simulink model "ABS_demo"  (R2018a)
settings: Solver=ode23t  StartTime=0.0  StopTime=20  RelTol=1e-3
values from neighbouring files (symbols this model uses):
  g = 9.81    [variables_values.m]
  I = 5    [variables_values.m]
  m = 75    [variables_values.m]
  R = 1.25    [variables_values.m]
  v0 = 44    [variables_values.m]
libraries: simulink x3
settings Model: Creator=Stephen Kingston  LastModifiedBy=adham
settings DataIOCC: ReturnWorkspaceOutputs=on
settings SFSimCC: SimUseLocalCustomCode=on
settings RTWCC: RTWUseLocalCustomCode=on

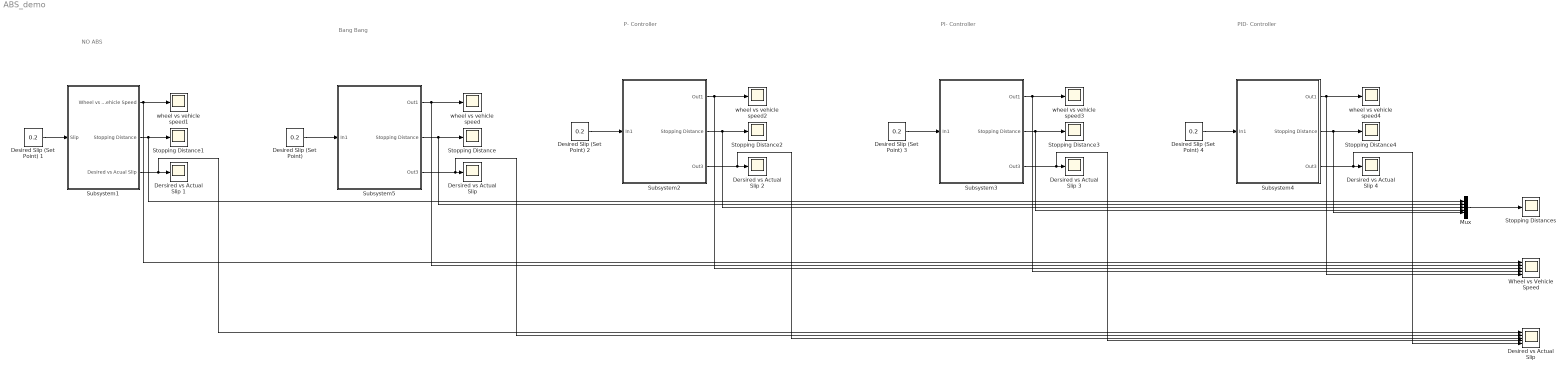
== system ABS_demo ==
  note: NO ABS
  note: Bang Bang
  note: P- Controller
  note: PI- Controller
  note: PID- Controller
  Dersired vs Actual Slip {,1..4} (5 alike) : Scope
  Desired Slip (Set Point) {,1..4} (5 alike) : Constant  Value=0.2
  Desired vs Actual Slip : Scope  NumInputPorts=5
  Mux : Mux  Inputs=5
  Stopping Distance{,1..4} (5 alike) : Scope
  Stopping Distances : Scope
  Subsystem1 : Subsystem
  Subsystem2 : Subsystem
  Subsystem3 : Subsystem
  Subsystem4 : Subsystem
  Subsystem5 : Subsystem
  Wheel vs Vehicle Speed : Scope  NumInputPorts=5
  wheel vs vehicle speed{,1..4} (5 alike) : Scope
  wires:
  Subsystem5/2(Stopping Distance) -> Mux/2, Stopping Distance/1
  "Desired Slip (Set Point) "/1 -> Subsystem5/1(In1)
  Subsystem1/2(Stopping Distance) -> Mux/1, Stopping Distance1/1
  Subsystem2/1(Out1) -> Wheel vs Vehicle Speed/3, wheel vs vehicle speed2/1
  Desired Slip (Set Point) 2/1 -> Subsystem2/1(In1)
  Desired Slip (Set Point) 3/1 -> Subsystem3/1(In1)
  Subsystem3/1(Out1) -> Wheel vs Vehicle Speed/4, wheel vs vehicle speed3/1
  Subsystem4/1(Out1) -> Wheel vs Vehicle Speed/5, wheel vs vehicle speed4/1
  Subsystem4/2(Stopping Distance) -> Mux/5, Stopping Distance4/1
  Desired Slip (Set Point) 4/1 -> Subsystem4/1(In1)
  Subsystem4/3(Out3) -> Desired vs Actual Slip/5, Dersired vs Actual Slip 4/1
  Mux/1 -> Stopping Distances/1
  Subsystem2/2(Stopping Distance) -> Mux/3, Stopping Distance2/1
  Subsystem3/2(Stopping Distance) -> Mux/4, Stopping Distance3/1
  Subsystem5/1(Out1) -> Wheel vs Vehicle Speed/2, wheel vs vehicle speed/1
  Subsystem1/1(Wheel vs Vehicle Speed) -> Wheel vs Vehicle Speed/1, wheel vs vehicle speed1/1
  Subsystem1/3(Desired vs Acual Slip) -> Desired vs Actual Slip/1, Dersired vs Actual Slip 1/1
  Subsystem5/3(Out3) -> Desired vs Actual Slip/2, "Dersired vs Actual Slip "/1
  Desired Slip (Set Point) 1/1 -> Subsystem1/1(Slip)
  Subsystem2/3(Out3) -> Desired vs Actual Slip/3, Dersired vs Actual Slip 2/1
  Subsystem3/3(Out3) -> Desired vs Actual Slip/4, Dersired vs Actual Slip 3/1

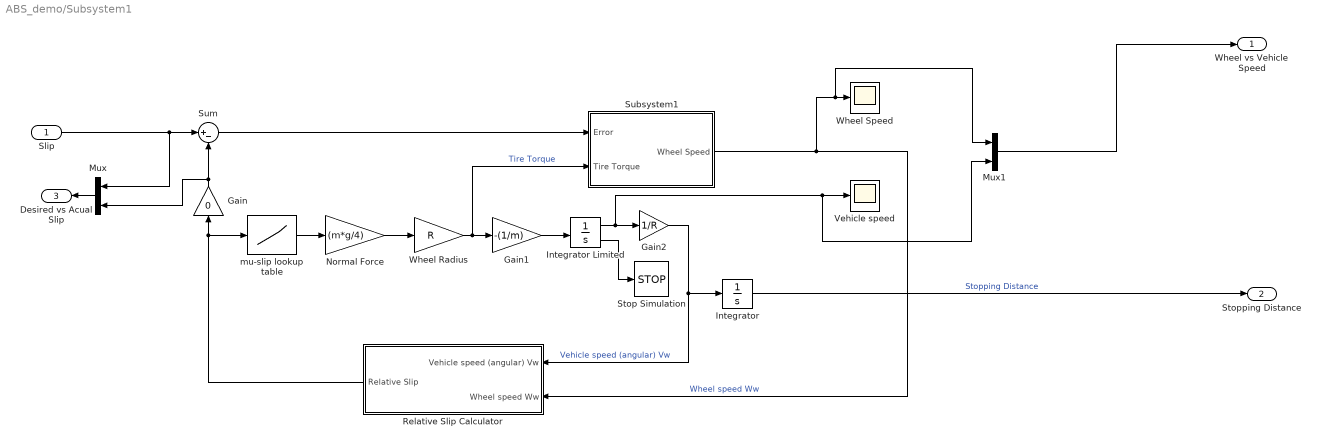
== system ABS_demo/Subsystem1 ==
  Slip : Inport
  Gain : Gain  Gain=0
  Gain1 : Gain  Gain=-(1/m)
  Gain2 : Gain  Gain=1/R
  Integrator : Integrator
  Integrator Limited : Integrator  InitialCondition=v0  LimitOutput=on  UpperSaturationLimit=1000  LowerSaturationLimit=0  ShowSaturationPort=on
  Mux : Mux  Inputs=2
  Mux1 : Mux  Inputs=2
  Normal Force : Gain  Gain=(m*g/4)
  Relative Slip Calculator : Subsystem
  Stop Simulation : Stop
  Subsystem1 : Subsystem
  Sum : Sum  Inputs=|+-
  Vehicle speed : Scope
  Wheel Radius : Gain  Gain=R
  Wheel Speed : Scope
  mu-slip lookup table : Lookup_n-D  NumberOfTableDimensions=1  BreakpointsForDimension1=[0,0.05,0.1,0.15,0.2,0.25,0.3,0.35,0.4,0.45,0.5,0.55,0.60,0.65,0.70,0.75,0.80,0.85,0.90,0.95,1]  Table=[0,0.4,0.8,0.97,1,0.98,0.96,0.94,0.92,0.9,0.88,0.855,0.83,0.81,0.79,0.77,0.75,0.73,0.72,0.71,0.7]  InternalRulePriority=Speed  RndMeth=Simplest  InputSameDT=on
  Wheel vs Vehicle Speed : Outport
  Stopping Distance : Outport  Port=2
  Desired vs Acual Slip : Outport  Port=3
  wires:
  Normal Force/1 -> Wheel Radius/1
  Subsystem1/1(Wheel Speed) -> Mux1/1, Wheel Speed/1, Relative Slip Calculator/2(Wheel speed Ww)  "Wheel speed Ww"
  Integrator Limited/1 -> Mux1/2, Vehicle speed/1, Gain2/1
  Gain/1 -> Mux/2, Sum/2
  Sum/1 -> Subsystem1/1(Error)
  Slip/1 -> Mux/1, Sum/1
  Integrator Limited/2 -> Stop Simulation/1
  Gain2/1 -> Relative Slip Calculator/1(Vehicle speed (angular) Vw), Integrator/1  "Vehicle speed (angular) Vw"
  mu-slip lookup table/1 -> Normal Force/1
  Wheel Radius/1 -> Gain1/1, Subsystem1/2(Tire Torque)  "Tire Torque"
  Gain1/1 -> Integrator Limited/1
  Relative Slip Calculator/1(Relative Slip) -> mu-slip lookup table/1, Gain/1
  Integrator/1 -> Stopping Distance/1  "Stopping Distance"
  Mux/1 -> Desired vs Acual Slip/1
  Mux1/1 -> Wheel vs Vehicle Speed/1

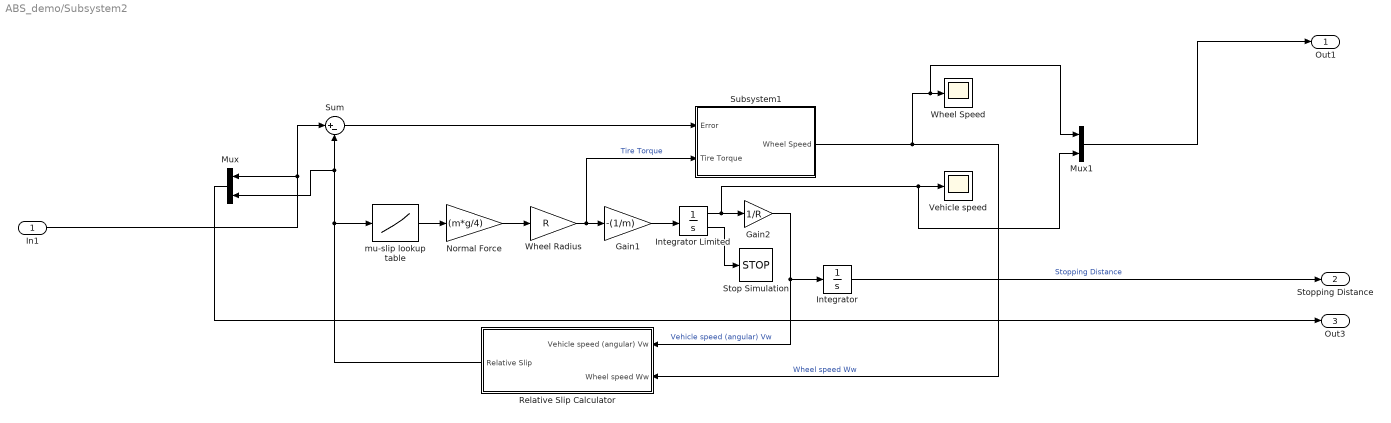
== system ABS_demo/Subsystem2 ==
  In1 : Inport
  Gain1 : Gain  Gain=-(1/m)
  Gain2 : Gain  Gain=1/R
  Integrator : Integrator
  Integrator Limited : Integrator  InitialCondition=v0  LimitOutput=on  UpperSaturationLimit=1000  LowerSaturationLimit=0  ShowSaturationPort=on
  Mux : Mux  Inputs=2
  Mux1 : Mux  Inputs=2
  Normal Force : Gain  Gain=(m*g/4)
  Relative Slip Calculator : Subsystem
  Stop Simulation : Stop
  Subsystem1 : Subsystem
  Sum : Sum  Inputs=|+-
  Vehicle speed : Scope
  Wheel Radius : Gain  Gain=R
  Wheel Speed : Scope
  mu-slip lookup table : Lookup_n-D  NumberOfTableDimensions=1  BreakpointsForDimension1=[0,0.05,0.1,0.15,0.2,0.25,0.3,0.35,0.4,0.45,0.5,0.55,0.60,0.65,0.70,0.75,0.80,0.85,0.90,0.95,1]  Table=[0,0.4,0.8,0.97,1,0.98,0.96,0.94,0.92,0.9,0.88,0.855,0.83,0.81,0.79,0.77,0.75,0.73,0.72,0.71,0.7]  InternalRulePriority=Speed  RndMeth=Simplest  InputSameDT=on
  Out1 : Outport
  Stopping Distance : Outport  Port=2
  Out3 : Outport  Port=3
  wires:
  Normal Force/1 -> Wheel Radius/1
  Subsystem1/1(Wheel Speed) -> Mux1/1, Wheel Speed/1, Relative Slip Calculator/2(Wheel speed Ww)  "Wheel speed Ww"
  Integrator Limited/1 -> Mux1/2, Vehicle speed/1, Gain2/1
  Relative Slip Calculator/1(Relative Slip) -> Mux/2, Sum/2, mu-slip lookup table/1
  Sum/1 -> Subsystem1/1(Error)
  In1/1 -> Sum/1, Mux/1
  Integrator Limited/2 -> Stop Simulation/1
  Gain2/1 -> Relative Slip Calculator/1(Vehicle speed (angular) Vw), Integrator/1  "Vehicle speed (angular) Vw"
  mu-slip lookup table/1 -> Normal Force/1
  Wheel Radius/1 -> Gain1/1, Subsystem1/2(Tire Torque)  "Tire Torque"
  Gain1/1 -> Integrator Limited/1
  Integrator/1 -> Stopping Distance/1  "Stopping Distance"
  Mux/1 -> Out3/1
  Mux1/1 -> Out1/1

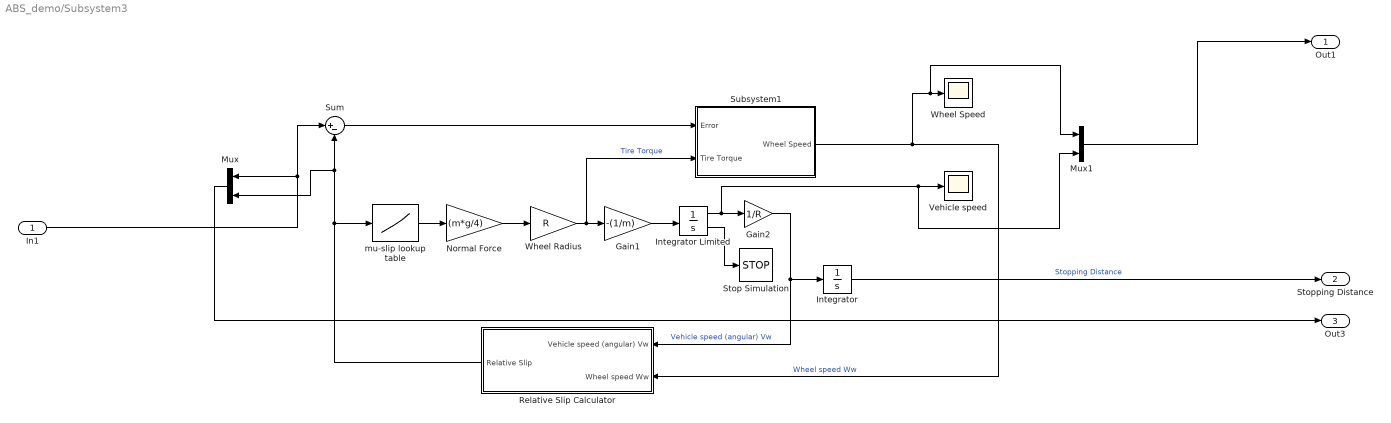
== system ABS_demo/Subsystem3 ==
  In1 : Inport
  Gain1 : Gain  Gain=-(1/m)
  Gain2 : Gain  Gain=1/R
  Integrator : Integrator
  Integrator Limited : Integrator  InitialCondition=v0  LimitOutput=on  UpperSaturationLimit=1000  LowerSaturationLimit=0  ShowSaturationPort=on
  Mux : Mux  Inputs=2
  Mux1 : Mux  Inputs=2
  Normal Force : Gain  Gain=(m*g/4)
  Relative Slip Calculator : Subsystem
  Stop Simulation : Stop
  Subsystem1 : Subsystem
  Sum : Sum  Inputs=|+-
  Vehicle speed : Scope
  Wheel Radius : Gain  Gain=R
  Wheel Speed : Scope
  mu-slip lookup table : Lookup_n-D  NumberOfTableDimensions=1  BreakpointsForDimension1=[0,0.05,0.1,0.15,0.2,0.25,0.3,0.35,0.4,0.45,0.5,0.55,0.60,0.65,0.70,0.75,0.80,0.85,0.90,0.95,1]  Table=[0,0.4,0.8,0.97,1,0.98,0.96,0.94,0.92,0.9,0.88,0.855,0.83,0.81,0.79,0.77,0.75,0.73,0.72,0.71,0.7]  InternalRulePriority=Speed  RndMeth=Simplest  InputSameDT=on
  Out1 : Outport
  Stopping Distance : Outport  Port=2
  Out3 : Outport  Port=3
  wires:
  Normal Force/1 -> Wheel Radius/1
  Subsystem1/1(Wheel Speed) -> Mux1/1, Wheel Speed/1, Relative Slip Calculator/2(Wheel speed Ww)  "Wheel speed Ww"
  Integrator Limited/1 -> Mux1/2, Vehicle speed/1, Gain2/1
  Relative Slip Calculator/1(Relative Slip) -> Mux/2, Sum/2, mu-slip lookup table/1
  Sum/1 -> Subsystem1/1(Error)
  In1/1 -> Sum/1, Mux/1
  Integrator Limited/2 -> Stop Simulation/1
  Gain2/1 -> Relative Slip Calculator/1(Vehicle speed (angular) Vw), Integrator/1  "Vehicle speed (angular) Vw"
  mu-slip lookup table/1 -> Normal Force/1
  Wheel Radius/1 -> Gain1/1, Subsystem1/2(Tire Torque)  "Tire Torque"
  Gain1/1 -> Integrator Limited/1
  Integrator/1 -> Stopping Distance/1  "Stopping Distance"
  Mux/1 -> Out3/1
  Mux1/1 -> Out1/1

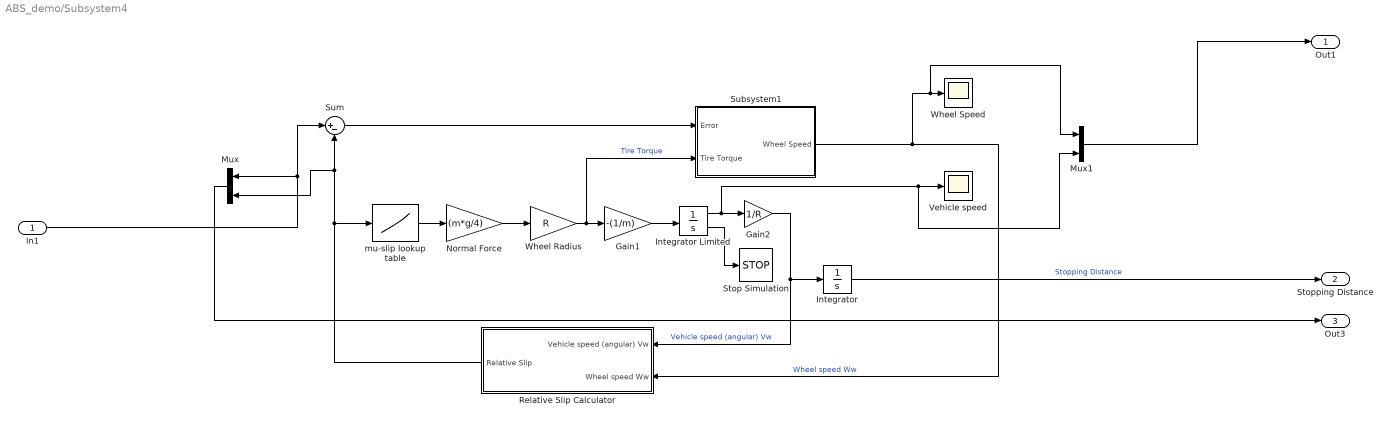
== system ABS_demo/Subsystem4 ==
  In1 : Inport
  Gain1 : Gain  Gain=-(1/m)
  Gain2 : Gain  Gain=1/R
  Integrator : Integrator
  Integrator Limited : Integrator  InitialCondition=v0  LimitOutput=on  UpperSaturationLimit=1000  LowerSaturationLimit=0  ShowSaturationPort=on
  Mux : Mux  Inputs=2
  Mux1 : Mux  Inputs=2
  Normal Force : Gain  Gain=(m*g/4)
  Relative Slip Calculator : Subsystem
  Stop Simulation : Stop
  Subsystem1 : Subsystem
  Sum : Sum  Inputs=|+-
  Vehicle speed : Scope
  Wheel Radius : Gain  Gain=R
  Wheel Speed : Scope
  mu-slip lookup table : Lookup_n-D  NumberOfTableDimensions=1  BreakpointsForDimension1=[0,0.05,0.1,0.15,0.2,0.25,0.3,0.35,0.4,0.45,0.5,0.55,0.60,0.65,0.70,0.75,0.80,0.85,0.90,0.95,1]  Table=[0,0.4,0.8,0.97,1,0.98,0.96,0.94,0.92,0.9,0.88,0.855,0.83,0.81,0.79,0.77,0.75,0.73,0.72,0.71,0.7]  InternalRulePriority=Speed  RndMeth=Simplest  InputSameDT=on
  Out1 : Outport
  Stopping Distance : Outport  Port=2
  Out3 : Outport  Port=3
  wires:
  Normal Force/1 -> Wheel Radius/1
  Subsystem1/1(Wheel Speed) -> Mux1/1, Wheel Speed/1, Relative Slip Calculator/2(Wheel speed Ww)  "Wheel speed Ww"
  Integrator Limited/1 -> Mux1/2, Vehicle speed/1, Gain2/1
  Relative Slip Calculator/1(Relative Slip) -> Mux/2, Sum/2, mu-slip lookup table/1
  Sum/1 -> Subsystem1/1(Error)
  In1/1 -> Sum/1, Mux/1
  Integrator Limited/2 -> Stop Simulation/1
  Gain2/1 -> Relative Slip Calculator/1(Vehicle speed (angular) Vw), Integrator/1  "Vehicle speed (angular) Vw"
  mu-slip lookup table/1 -> Normal Force/1
  Wheel Radius/1 -> Gain1/1, Subsystem1/2(Tire Torque)  "Tire Torque"
  Gain1/1 -> Integrator Limited/1
  Integrator/1 -> Stopping Distance/1  "Stopping Distance"
  Mux/1 -> Out3/1
  Mux1/1 -> Out1/1

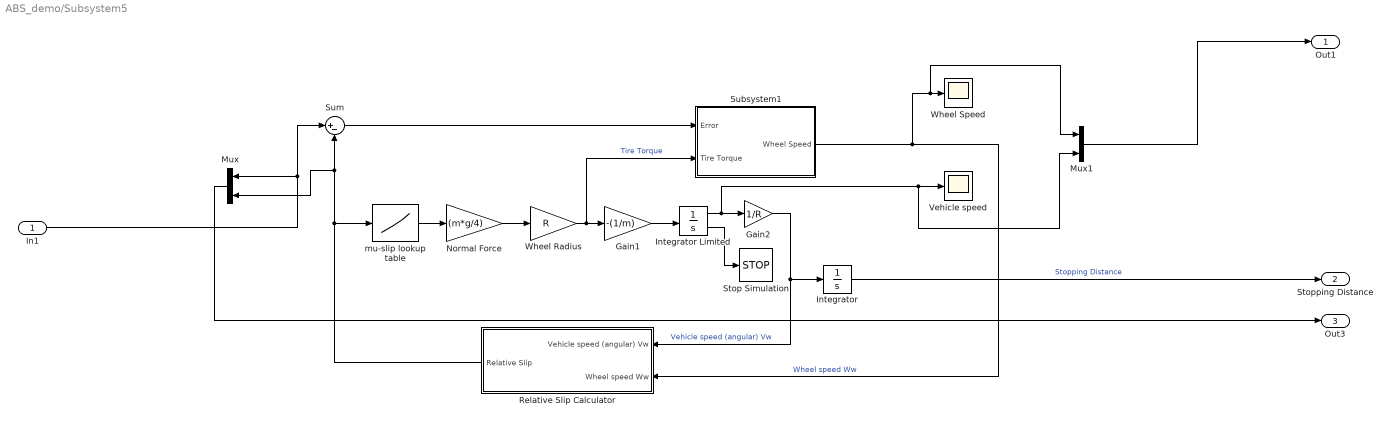
== system ABS_demo/Subsystem5 ==
  In1 : Inport
  Gain1 : Gain  Gain=-(1/m)
  Gain2 : Gain  Gain=1/R
  Integrator : Integrator
  Integrator Limited : Integrator  InitialCondition=v0  LimitOutput=on  UpperSaturationLimit=1000  LowerSaturationLimit=0  ShowSaturationPort=on
  Mux : Mux  Inputs=2
  Mux1 : Mux  Inputs=2
  Normal Force : Gain  Gain=(m*g/4)
  Relative Slip Calculator : Subsystem
  Stop Simulation : Stop
  Subsystem1 : Subsystem
  Sum : Sum  Inputs=|+-
  Vehicle speed : Scope
  Wheel Radius : Gain  Gain=R
  Wheel Speed : Scope
  mu-slip lookup table : Lookup_n-D  NumberOfTableDimensions=1  BreakpointsForDimension1=[0,0.05,0.1,0.15,0.2,0.25,0.3,0.35,0.4,0.45,0.5,0.55,0.60,0.65,0.70,0.75,0.80,0.85,0.90,0.95,1]  Table=[0,0.4,0.8,0.97,1,0.98,0.96,0.94,0.92,0.9,0.88,0.855,0.83,0.81,0.79,0.77,0.75,0.73,0.72,0.71,0.7]  InternalRulePriority=Speed  RndMeth=Simplest  InputSameDT=on
  Out1 : Outport
  Stopping Distance : Outport  Port=2
  Out3 : Outport  Port=3
  wires:
  Normal Force/1 -> Wheel Radius/1
  Subsystem1/1(Wheel Speed) -> Mux1/1, Wheel Speed/1, Relative Slip Calculator/2(Wheel speed Ww)  "Wheel speed Ww"
  Integrator Limited/1 -> Mux1/2, Vehicle speed/1, Gain2/1
  Relative Slip Calculator/1(Relative Slip) -> Mux/2, Sum/2, mu-slip lookup table/1
  Sum/1 -> Subsystem1/1(Error)
  In1/1 -> Sum/1, Mux/1
  Integrator Limited/2 -> Stop Simulation/1
  Gain2/1 -> Relative Slip Calculator/1(Vehicle speed (angular) Vw), Integrator/1  "Vehicle speed (angular) Vw"
  mu-slip lookup table/1 -> Normal Force/1
  Wheel Radius/1 -> Gain1/1, Subsystem1/2(Tire Torque)  "Tire Torque"
  Gain1/1 -> Integrator Limited/1
  Integrator/1 -> Stopping Distance/1  "Stopping Distance"
  Mux/1 -> Out3/1
  Mux1/1 -> Out1/1

== system ABS_demo/Subsystem1/Relative Slip Calculator ==
  Vehicle speed (angular) Vw : Inport
  Wheel speed Ww : Inport  Port=2
  Constant : Constant
  Divide : Product  Inputs=/*
  Sum1 : Sum  Inputs=|+-
  Relative Slip : Outport
  wires:
  Divide/1 -> Sum1/2
  Sum1/1 -> Relative Slip/1
  Constant/1 -> Sum1/1
  Wheel speed Ww/1 -> Divide/2
  Vehicle speed (angular) Vw/1 -> Divide/1

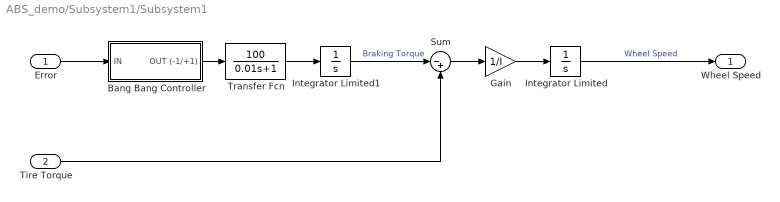
== system ABS_demo/Subsystem1/Subsystem1 ==
  Error : Inport
  Tire Torque : Inport  Port=2
  Bang Bang Controller : Subsystem
  Gain : Gain  Gain=1/I
  Integrator Limited : Integrator  InitialCondition=v0/R  LimitOutput=on  UpperSaturationLimit=1000  LowerSaturationLimit=0
  Integrator Limited1 : Integrator  LimitOutput=on  UpperSaturationLimit=1500  LowerSaturationLimit=0
  Sum : Sum  Inputs=|-+
  Transfer Fcn : TransferFcn  Numerator=[100]  Denominator=[0.01 1]
  Wheel Speed : Outport
  wires:
  Sum/1 -> Gain/1
  Transfer Fcn/1 -> Integrator Limited1/1
  Gain/1 -> Integrator Limited/1
  Integrator Limited/1 -> Wheel Speed/1  "Wheel Speed"
  Integrator Limited1/1 -> Sum/1  "Braking Torque"
  Bang Bang Controller/1(OUT (-1/+1)) -> Transfer Fcn/1
  Tire Torque/1 -> Sum/2
  Error/1 -> Bang Bang Controller/1(IN)

== system ABS_demo/Subsystem2/Relative Slip Calculator ==
  Vehicle speed (angular) Vw : Inport
  Wheel speed Ww : Inport  Port=2
  Constant : Constant
  Divide : Product  Inputs=/*
  Sum1 : Sum  Inputs=|+-
  Relative Slip : Outport
  wires:
  Divide/1 -> Sum1/2
  Sum1/1 -> Relative Slip/1
  Constant/1 -> Sum1/1
  Wheel speed Ww/1 -> Divide/2
  Vehicle speed (angular) Vw/1 -> Divide/1

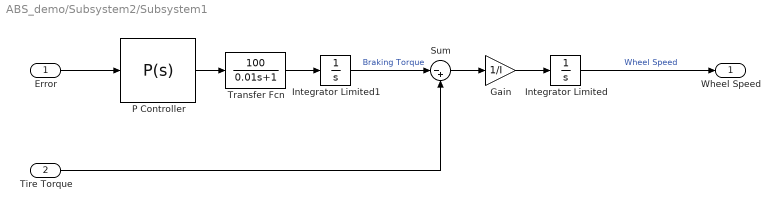
== system ABS_demo/Subsystem2/Subsystem1 ==
  Error : Inport
  Tire Torque : Inport  Port=2
  Gain : Gain  Gain=1/I
  Integrator Limited : Integrator  InitialCondition=v0/R  LimitOutput=on  UpperSaturationLimit=1000  LowerSaturationLimit=0
  Integrator Limited1 : Integrator  LimitOutput=on  UpperSaturationLimit=1500  LowerSaturationLimit=0
  P Controller : simulink/Continuous/PID Controller  Controller=P  TimeDomain=Continuous-time  SampleTime=-1  IntegratorMethod=Forward Euler  FilterMethod=Forward Euler  Form=Parallel  UseFilter=on  ControllerParametersSource=internal  P=30534.7737654381  I=0  D=0  N=0  InitialConditionSource=internal  InitialConditionForIntegrator=0  InitialConditionForFilter=0  ExternalReset=none  LimitOutput=off  UpperSaturationLimit=inf  LowerSaturationLimit=-inf  LinearizeAsGain=on  AntiWindupMode=none  Kb=1  TrackingMode=off  Kt=1  PParamMin=[]  PParamMax=[]  IParamMin=[]  IParamMax=[]  DParamMin=[]  DParamMax=[]  NParamMin=[]  NParamMax=[]  KbParamMin=[]  KbParamMax=[]  KtParamMin=[]  KtParamMax=[]  POutMin=[]  POutMax=[]  IOutMin=[]  IOutMax=[]  DOutMin=[]  DOutMax=[]  NOutMin=[]  NOutMax=[]  KbOutMin=[]  KbOutMax=[]  KtOutMin=[]  KtOutMax=[]  IntegratorOutMin=[]  IntegratorOutMax=[]  FilterOutMin=[]  FilterOutMax=[]  SumOutMin=[]  SumOutMax=[]  SumI1OutMin=[]  SumI1OutMax=[]  SumI2OutMin=[]  SumI2OutMax=[]  SumI3OutMin=[]  SumI3OutMax=[]  SumDOutMin=[]  SumDOutMax=[]  SaturationOutMin=[]  SaturationOutMax=[]  IntegratorContinuousStateAttributes=''  IntegratorStateMustResolveToSignalObject=off  IntegratorRTWStateStorageClass=Auto  FilterContinuousStateAttributes=''  FilterStateMustResolveToSignalObject=off  FilterRTWStateStorageClass=Auto  DifferentiatorICPrevScaledInput=0  DifferentiatorOutMin=[]  DifferentiatorOutMax=[]  FilterDiffOutCoefMin=[]  FilterDiffOutCoefMax=[]  SumDenOutMin=[]  SumDenOutMax=[]  SumNumOutMin=[]  SumNumOutMax=[]  ReciprocalOutMin=[]  ReciprocalOutMax=[]  DivideOutMin=[]  DivideOutMax=[]  TunerSelectOption=Transfer Function Based (PID Tuner App)
  Sum : Sum  Inputs=|-+
  Transfer Fcn : TransferFcn  Numerator=[100]  Denominator=[0.01 1]
  Wheel Speed : Outport
  wires:
  Sum/1 -> Gain/1
  Transfer Fcn/1 -> Integrator Limited1/1
  Gain/1 -> Integrator Limited/1
  Integrator Limited/1 -> Wheel Speed/1  "Wheel Speed"
  Integrator Limited1/1 -> Sum/1  "Braking Torque"
  P Controller/1 -> Transfer Fcn/1
  Tire Torque/1 -> Sum/2
  Error/1 -> P Controller/1

== system ABS_demo/Subsystem3/Relative Slip Calculator ==
  Vehicle speed (angular) Vw : Inport
  Wheel speed Ww : Inport  Port=2
  Constant : Constant
  Divide : Product  Inputs=/*
  Sum1 : Sum  Inputs=|+-
  Relative Slip : Outport
  wires:
  Divide/1 -> Sum1/2
  Sum1/1 -> Relative Slip/1
  Constant/1 -> Sum1/1
  Wheel speed Ww/1 -> Divide/2
  Vehicle speed (angular) Vw/1 -> Divide/1

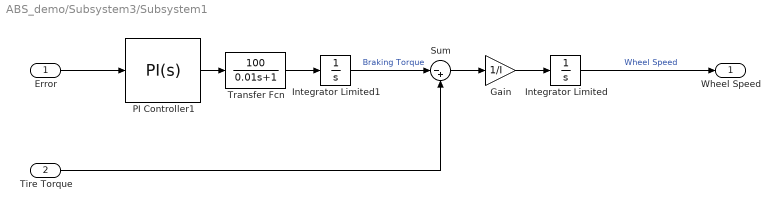
== system ABS_demo/Subsystem3/Subsystem1 ==
  Error : Inport
  Tire Torque : Inport  Port=2
  Gain : Gain  Gain=1/I
  Integrator Limited : Integrator  InitialCondition=v0/R  LimitOutput=on  UpperSaturationLimit=1000  LowerSaturationLimit=0
  Integrator Limited1 : Integrator  LimitOutput=on  UpperSaturationLimit=1500  LowerSaturationLimit=0
  PI Controller1 : simulink/Continuous/PID Controller  Controller=PI  TimeDomain=Continuous-time  SampleTime=-1  IntegratorMethod=Forward Euler  FilterMethod=Forward Euler  Form=Parallel  UseFilter=on  ControllerParametersSource=internal  P=30534.7737654381  I=1487437.43001802  D=0  N=0  InitialConditionSource=internal  InitialConditionForIntegrator=0  InitialConditionForFilter=0  ExternalReset=none  LimitOutput=off  UpperSaturationLimit=inf  LowerSaturationLimit=-inf  LinearizeAsGain=on  AntiWindupMode=none  Kb=1  TrackingMode=off  Kt=1  PParamMin=[]  PParamMax=[]  IParamMin=[]  IParamMax=[]  DParamMin=[]  DParamMax=[]  NParamMin=[]  NParamMax=[]  KbParamMin=[]  KbParamMax=[]  KtParamMin=[]  KtParamMax=[]  POutMin=[]  POutMax=[]  IOutMin=[]  IOutMax=[]  DOutMin=[]  DOutMax=[]  NOutMin=[]  NOutMax=[]  KbOutMin=[]  KbOutMax=[]  KtOutMin=[]  KtOutMax=[]  IntegratorOutMin=[]  IntegratorOutMax=[]  FilterOutMin=[]  FilterOutMax=[]  SumOutMin=[]  SumOutMax=[]  SumI1OutMin=[]  SumI1OutMax=[]  SumI2OutMin=[]  SumI2OutMax=[]  SumI3OutMin=[]  SumI3OutMax=[]  SumDOutMin=[]  SumDOutMax=[]  SaturationOutMin=[]  SaturationOutMax=[]  IntegratorContinuousStateAttributes=''  IntegratorStateMustResolveToSignalObject=off  IntegratorRTWStateStorageClass=Auto  FilterContinuousStateAttributes=''  FilterStateMustResolveToSignalObject=off  FilterRTWStateStorageClass=Auto  DifferentiatorICPrevScaledInput=0  DifferentiatorOutMin=[]  DifferentiatorOutMax=[]  FilterDiffOutCoefMin=[]  FilterDiffOutCoefMax=[]  SumDenOutMin=[]  SumDenOutMax=[]  SumNumOutMin=[]  SumNumOutMax=[]  ReciprocalOutMin=[]  ReciprocalOutMax=[]  DivideOutMin=[]  DivideOutMax=[]  TunerSelectOption=Transfer Function Based (PID Tuner App)
  Sum : Sum  Inputs=|-+
  Transfer Fcn : TransferFcn  Numerator=[100]  Denominator=[0.01 1]
  Wheel Speed : Outport
  wires:
  Sum/1 -> Gain/1
  Transfer Fcn/1 -> Integrator Limited1/1
  Gain/1 -> Integrator Limited/1
  Integrator Limited/1 -> Wheel Speed/1  "Wheel Speed"
  Integrator Limited1/1 -> Sum/1  "Braking Torque"
  PI Controller1/1 -> Transfer Fcn/1
  Tire Torque/1 -> Sum/2
  Error/1 -> PI Controller1/1

== system ABS_demo/Subsystem4/Relative Slip Calculator ==
  Vehicle speed (angular) Vw : Inport
  Wheel speed Ww : Inport  Port=2
  Constant : Constant
  Divide : Product  Inputs=/*
  Sum1 : Sum  Inputs=|+-
  Relative Slip : Outport
  wires:
  Divide/1 -> Sum1/2
  Sum1/1 -> Relative Slip/1
  Constant/1 -> Sum1/1
  Wheel speed Ww/1 -> Divide/2
  Vehicle speed (angular) Vw/1 -> Divide/1

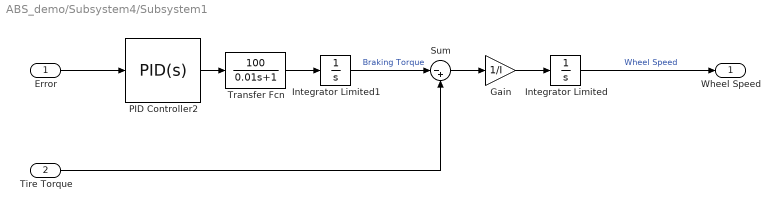
== system ABS_demo/Subsystem4/Subsystem1 ==
  Error : Inport
  Tire Torque : Inport  Port=2
  Gain : Gain  Gain=1/I
  Integrator Limited : Integrator  InitialCondition=v0/R  LimitOutput=on  UpperSaturationLimit=1000  LowerSaturationLimit=0
  Integrator Limited1 : Integrator  LimitOutput=on  UpperSaturationLimit=1500  LowerSaturationLimit=0
  PID Controller2 : simulink/Continuous/PID Controller  Controller=PID  TimeDomain=Continuous-time  SampleTime=-1  IntegratorMethod=Forward Euler  FilterMethod=Forward Euler  Form=Parallel  UseFilter=on  ControllerParametersSource=internal  P=30534.7737654381  I=1487437.43001802  D=43.0572758151789  N=0  InitialConditionSource=internal  InitialConditionForIntegrator=0  InitialConditionForFilter=0  ExternalReset=none  LimitOutput=off  UpperSaturationLimit=inf  LowerSaturationLimit=-inf  LinearizeAsGain=on  AntiWindupMode=none  Kb=1  TrackingMode=off  Kt=1  PParamMin=[]  PParamMax=[]  IParamMin=[]  IParamMax=[]  DParamMin=[]  DParamMax=[]  NParamMin=[]  NParamMax=[]  KbParamMin=[]  KbParamMax=[]  KtParamMin=[]  KtParamMax=[]  POutMin=[]  POutMax=[]  IOutMin=[]  IOutMax=[]  DOutMin=[]  DOutMax=[]  NOutMin=[]  NOutMax=[]  KbOutMin=[]  KbOutMax=[]  KtOutMin=[]  KtOutMax=[]  IntegratorOutMin=[]  IntegratorOutMax=[]  FilterOutMin=[]  FilterOutMax=[]  SumOutMin=[]  SumOutMax=[]  SumI1OutMin=[]  SumI1OutMax=[]  SumI2OutMin=[]  SumI2OutMax=[]  SumI3OutMin=[]  SumI3OutMax=[]  SumDOutMin=[]  SumDOutMax=[]  SaturationOutMin=[]  SaturationOutMax=[]  IntegratorContinuousStateAttributes=''  IntegratorStateMustResolveToSignalObject=off  IntegratorRTWStateStorageClass=Auto  FilterContinuousStateAttributes=''  FilterStateMustResolveToSignalObject=off  FilterRTWStateStorageClass=Auto  DifferentiatorICPrevScaledInput=0  DifferentiatorOutMin=[]  DifferentiatorOutMax=[]  FilterDiffOutCoefMin=[]  FilterDiffOutCoefMax=[]  SumDenOutMin=[]  SumDenOutMax=[]  SumNumOutMin=[]  SumNumOutMax=[]  ReciprocalOutMin=[]  ReciprocalOutMax=[]  DivideOutMin=[]  DivideOutMax=[]  TunerSelectOption=Transfer Function Based (PID Tuner App)
  Sum : Sum  Inputs=|-+
  Transfer Fcn : TransferFcn  Numerator=[100]  Denominator=[0.01 1]
  Wheel Speed : Outport
  wires:
  Sum/1 -> Gain/1
  Transfer Fcn/1 -> Integrator Limited1/1
  Gain/1 -> Integrator Limited/1
  Integrator Limited/1 -> Wheel Speed/1  "Wheel Speed"
  Integrator Limited1/1 -> Sum/1  "Braking Torque"
  PID Controller2/1 -> Transfer Fcn/1
  Tire Torque/1 -> Sum/2
  Error/1 -> PID Controller2/1

== system ABS_demo/Subsystem5/Relative Slip Calculator ==
  Vehicle speed (angular) Vw : Inport
  Wheel speed Ww : Inport  Port=2
  Constant : Constant
  Divide : Product  Inputs=/*
  Sum1 : Sum  Inputs=|+-
  Relative Slip : Outport
  wires:
  Divide/1 -> Sum1/2
  Sum1/1 -> Relative Slip/1
  Constant/1 -> Sum1/1
  Wheel speed Ww/1 -> Divide/2
  Vehicle speed (angular) Vw/1 -> Divide/1

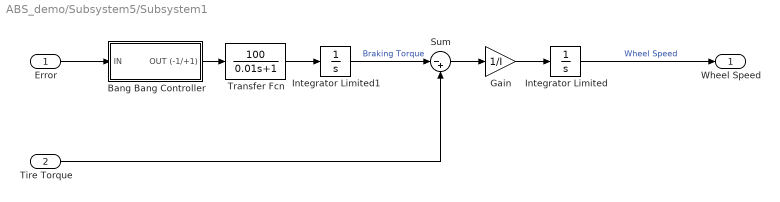
== system ABS_demo/Subsystem5/Subsystem1 ==
  Error : Inport
  Tire Torque : Inport  Port=2
  Bang Bang Controller : Subsystem
  Gain : Gain  Gain=1/I
  Integrator Limited : Integrator  InitialCondition=v0/R  LimitOutput=on  UpperSaturationLimit=1000  LowerSaturationLimit=0
  Integrator Limited1 : Integrator  LimitOutput=on  UpperSaturationLimit=1500  LowerSaturationLimit=0
  Sum : Sum  Inputs=|-+
  Transfer Fcn : TransferFcn  Numerator=[100]  Denominator=[0.01 1]
  Wheel Speed : Outport
  wires:
  Sum/1 -> Gain/1
  Transfer Fcn/1 -> Integrator Limited1/1
  Gain/1 -> Integrator Limited/1
  Integrator Limited/1 -> Wheel Speed/1  "Wheel Speed"
  Integrator Limited1/1 -> Sum/1  "Braking Torque"
  Bang Bang Controller/1(OUT (-1/+1)) -> Transfer Fcn/1
  Tire Torque/1 -> Sum/2
  Error/1 -> Bang Bang Controller/1(IN)

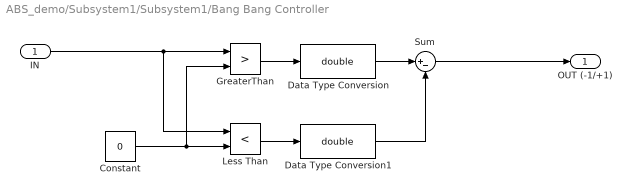
== system ABS_demo/Subsystem1/Subsystem1/Bang Bang Controller ==
  IN : Inport
  Constant : Constant  Value=0
  Data Type Conversion : DataTypeConversion  OutDataTypeStr=double  RndMeth=Zero
  Data Type Conversion1 : DataTypeConversion  OutDataTypeStr=double  RndMeth=Zero
  GreaterThan : RelationalOperator  Operator=>  OutDataTypeStr=boolean  RndMeth=Simplest
  Less Than : RelationalOperator  Operator=<  OutDataTypeStr=boolean  RndMeth=Simplest
  Sum : Sum  Inputs=|+-
  OUT (-1/+1) : Outport
  wires:
  Sum/1 -> OUT (-1/+1)/1
  Data Type Conversion/1 -> Sum/1
  Constant/1 -> GreaterThan/2, Less Than/2
  IN/1 -> Less Than/1, GreaterThan/1
  Data Type Conversion1/1 -> Sum/2
  GreaterThan/1 -> Data Type Conversion/1
  Less Than/1 -> Data Type Conversion1/1

== system ABS_demo/Subsystem5/Subsystem1/Bang Bang Controller ==
  IN : Inport
  Constant : Constant  Value=0
  Data Type Conversion : DataTypeConversion  OutDataTypeStr=double  RndMeth=Zero
  Data Type Conversion1 : DataTypeConversion  OutDataTypeStr=double  RndMeth=Zero
  GreaterThan : RelationalOperator  Operator=>  OutDataTypeStr=boolean  RndMeth=Simplest
  Less Than : RelationalOperator  Operator=<  OutDataTypeStr=boolean  RndMeth=Simplest
  Sum : Sum  Inputs=|+-
  OUT (-1/+1) : Outport
  wires:
  Sum/1 -> OUT (-1/+1)/1
  Data Type Conversion/1 -> Sum/1
  Constant/1 -> GreaterThan/2, Less Than/2
  IN/1 -> Less Than/1, GreaterThan/1
  Data Type Conversion1/1 -> Sum/2
  GreaterThan/1 -> Data Type Conversion/1
  Less Than/1 -> Data Type Conversion1/1
